simulink model "sun_seeking_solar_panel"  (R2023a)
settings: Solver=VariableStepAuto  StartTime=0.0  StopTime=10.0  RelTol=1e-3
undefined symbols (not defined in the file): J, K_d, K_f, K_g, K_t, L, R
libraries: slpidlib x1
settings Model: Creator=HP 1040G3 ci7  LastModifiedBy=HP 1040G3 ci7

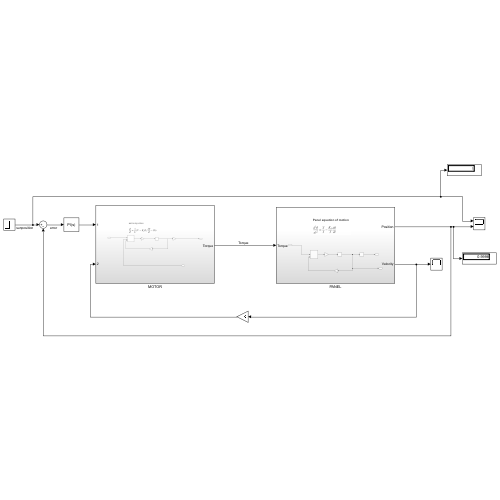
[thumbnail: Simulink's stored preview of the top-level diagram]
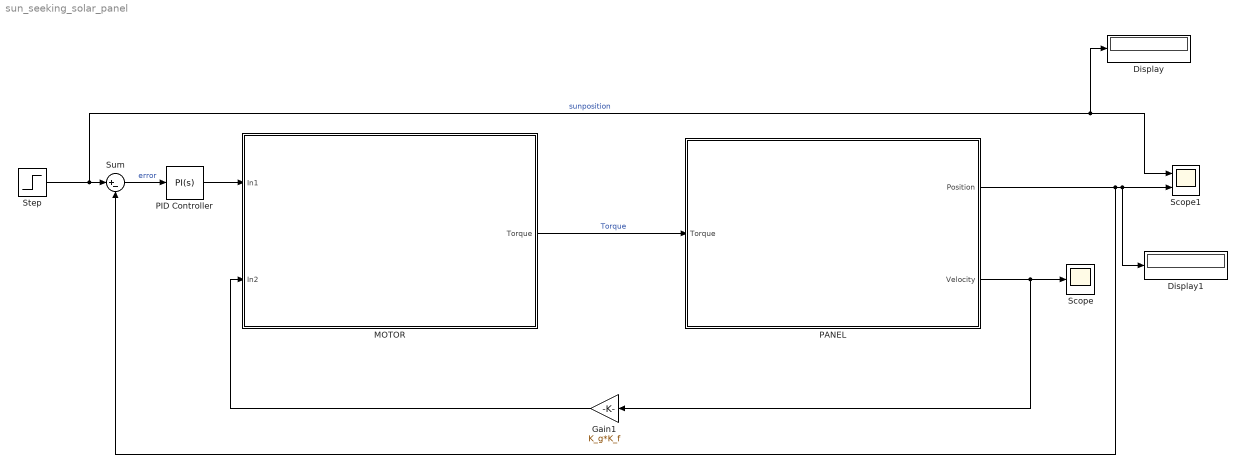
== system sun_seeking_solar_panel ==
  Display : Display
  Display1 : Display
  Gain1 : Gain  Gain=K_g*K_f
  MOTOR : Subsystem
  PANEL : Subsystem
  PID Controller : slpidlib/PID Controller  Controller=PI  Form=Parallel  TimeDomain=Continuous-time  UseExternalTs=off  SampleTime=-1  IntegratorMethod=Forward Euler  FilterMethod=Forward Euler  ControllerParametersSource=internal  P=240  I=180  UseKiTs=off  D=0  N=100  UseFilter=on  TunerSelectOption=Transfer Function Based (PID Tuner App)  InitialConditionSource=internal  InitialConditionForIntegrator=0  InitialConditionForFilter=0  DifferentiatorICPrevScaledInput=0  ExternalReset=none  TrackingMode=off  Kt=1  LimitOutput=off  SatLimitsSource=internal  UpperSaturationLimit=inf  LowerSaturationLimit=-inf  LinearizeAsGain=on  AntiWindupMode=none  Kb=1  LimitIntegrator=off  UpperIntegratorSaturationLimit=inf  LowerIntegratorSaturationLimit=-inf  POutMin=[]  POutMax=[]  IOutMin=[]  IOutMax=[]  DOutMin=[]  DOutMax=[]  NOutMin=[]  NOutMax=[]  SumOutMin=[]  SumOutMax=[]  SaturationOutMin=[]  SaturationOutMax=[]  PParamMin=[]  PParamMax=[]  IParamMin=[]  IParamMax=[]  DParamMin=[]  DParamMax=[]  NParamMin=[]  NParamMax=[]  KbParamMin=[]  KbParamMax=[]  KtParamMin=[]  KtParamMax=[]  KbOutMin=[]  KbOutMax=[]  KtOutMin=[]  KtOutMax=[]  IntegratorOutMin=[]  IntegratorOutMax=[]  FilterOutMin=[]  FilterOutMax=[]  SumI1OutMin=[]  SumI1OutMax=[]  SumI2OutMin=[]  SumI2OutMax=[]  SumI3OutMin=[]  SumI3OutMax=[]  SumI4OutMin=[]  SumI4OutMax=[]  SumDOutMin=[]  SumDOutMax=[]  DifferentiatorOutMin=[]  DifferentiatorOutMax=[]  FilterDiffOutCoefMin=[]  FilterDiffOutCoefMax=[]  ReciprocalOutMin=[]  ReciprocalOutMax=[]  SumDenOutMin=[]  SumDenOutMax=[]  SumNumOutMin=[]  SumNumOutMax=[]  DivideOutMin=[]  DivideOutMax=[]  UdiffTsProdOutMin=[]  UdiffTsProdOutMax=[]  NTsProdOutMin=[]  NTsProdOutMax=[]  UintegralTsProdOutMin=[]  UintegralTsProdOutMax=[]  UngainTsProdOutMin=[]  UngainTsProdOutMax=[]  ClampingZeroOutDataTypeStr=Inherit: Inherit via back propagation  ClampingZeroOutMin=[]  ClampingZeroOutMax=[]  FilterDenConstantOutDataTypeStr=Inherit: Inherit via back propagation  FilterDenConstantOutMin=[]  FilterDenConstantOutMax=[]  PCopyOutDataTypeStr=Inherit: Inherit via back propagation  PCopyOutMin=[]  PCopyOutMax=[]  NCopyOutDataTypeStr=Inherit: Inherit via back propagation  NCopyOutMin=[]  NCopyOutMax=[]  IntegratorContinuousStateAttributes=''  IntegratorStateMustResolveToSignalObject=off  IntegratorRTWStateStorageClass=Auto  FilterContinuousStateAttributes=''  FilterStateMustResolveToSignalObject=off  FilterRTWStateStorageClass=Auto  ParallelPVariant=InternalParameters  IdealPVariant=Disabled  IVariant=InternalParameters  DVariant=Disabled  IntegratorVariant=Continuous  SatVariant=Disabled  AWVariant=Passthrough  PCopyVariant=Disabled  TRVariant=Disabled  FdbkBlocksVariant=Forward  IdealPFdbkVariant=Disabled  SatFdbkVariant=Disabled  DerivativeFilterVariant=Disabled  NVariant=Disabled  NCopyVariant=Disabled_SignalSpec  FilterICVariant=Disabled  IntegratorICVariant=InternalICs  ExternalResetVariant=Disabled  TRSumVariant=Passthrough  SumFdbkVariant=Disabled  SumVariant=Sum_PI  TsampFilterVariant=InternalTs  TsampNgainVariant=Passthrough  TsampIntegralVariant=Disabled_SignalSpec  ExternalSaturationOutDataTypeStr=Inherit: Same as second input
  Scope : Scope
  Scope1 : Scope  NumInputPorts=2
  Step : Step  SampleTime=0
  Sum : Sum  Inputs=|+-
  wires:
  Gain1/1 -> MOTOR/2(In2)
  MOTOR/1(Torque) -> PANEL/1(Torque)  "Torque"
  PANEL/1(Position) -> Scope1/2, Display1/1, Sum/2
  PANEL/2(Velocity) -> Gain1/1, Scope/1
  Step/1 -> Display/1, Scope1/1, Sum/1  "sunposition"
  PID Controller/1 -> MOTOR/1(In1)
  Sum/1 -> PID Controller/1  "error"

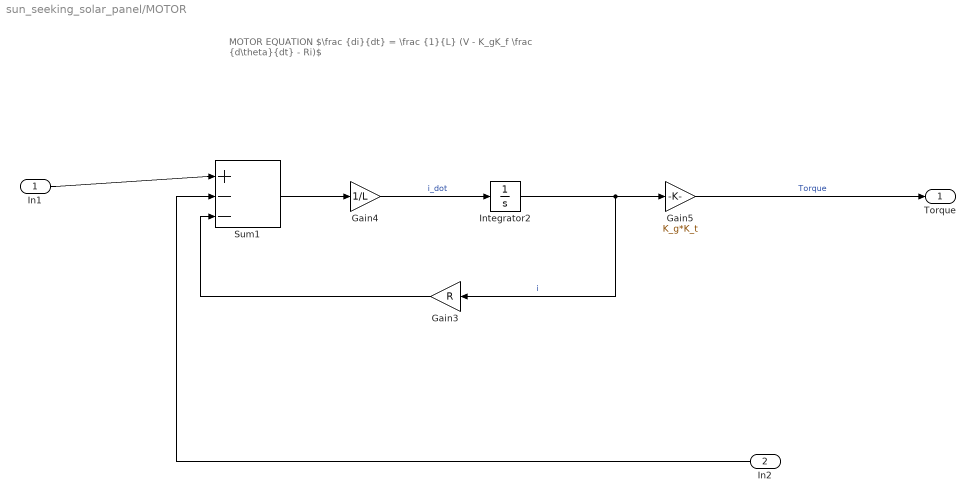
== system sun_seeking_solar_panel/MOTOR ==
  note: MOTOR EQUATION
      |
      | $\frac {di}{dt} = \frac {1}{L} (V - K_gK_f \frac {d\theta}{dt} - Ri)$
  In1 : Inport
  In2 : Inport  Port=2
  Gain3 : Gain  Gain=R
  Gain4 : Gain  Gain=1/L
  Gain5 : Gain  Gain=K_g*K_t
  Integrator2 : Integrator
  Sum1 : Sum  Inputs=|+--
  Torque : Outport
  wires:
  In2/1 -> Sum1/2
  In1/1 -> Sum1/1
  Gain3/1 -> Sum1/3
  Gain4/1 -> Integrator2/1  "i_dot"
  Integrator2/1 -> Gain5/1, Gain3/1  "i"
  Sum1/1 -> Gain4/1
  Gain5/1 -> Torque/1  "Torque"

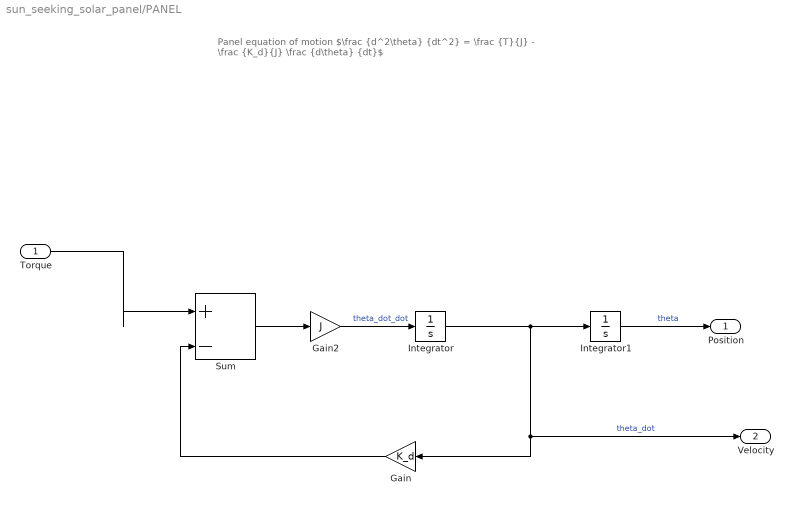
== system sun_seeking_solar_panel/PANEL ==
  note: Panel equation of motion
      |
      | $\frac {d^2\theta} {dt^2} = \frac {T}{J} - \frac {K_d}{J} \frac {d\theta} {dt}$
  Torque : Inport
  Gain : Gain  Gain=K_d
  Gain2 : Gain  Gain=J
  Integrator : Integrator
  Integrator1 : Integrator
  Sum : Sum  Inputs=|+-
  Position : Outport
  Velocity : Outport  Port=2
  wires:
  Integrator1/1 -> Position/1  "theta"
  Integrator/1 -> Integrator1/1, Velocity/1, Gain/1  "theta_dot"
  Torque/1 -> Sum/1
  Sum/1 -> Gain2/1
  Gain/1 -> Sum/2
  Gain2/1 -> Integrator/1  "theta_dot_dot"
